simulink model "CPWalker_NAO_simulation"  (R2021b)
settings: Solver=FixedStepDiscrete  StartTime=0.0  StopTime=inf  FixedStep=0.01  RelTol=1e-3
libraries: slrealtimeutilitieslib x1, slrealtimeiplib x1, dspnetwork x1
settings Model: Creator=Julio Lora  LastModifiedBy=mtmau
settings SolverCC: AlgebraicLoopSolver=TrustRegion
settings DataIOCC: ReturnWorkspaceOutputs=off
settings DebuggingCC: SFMachineParentedDataDiag=warning  ArithmeticOperatorsInVariantConditions=warning
settings SFSimCC: SimUseLocalCustomCode=off  CustomCodeUndefinedFunction=UseInterfaceOnly
settings RTWCC: RTWUseLocalCustomCode=off

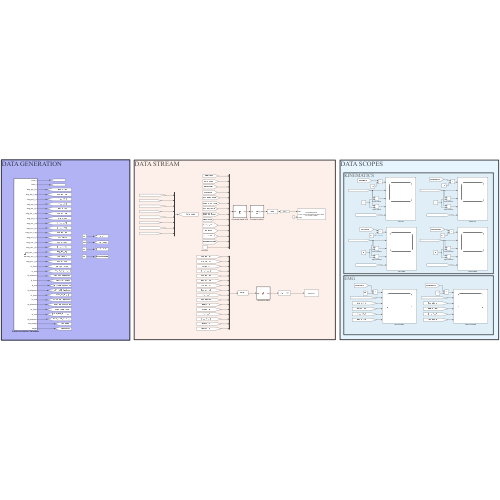
[thumbnail: Simulink's stored preview of the top-level diagram]
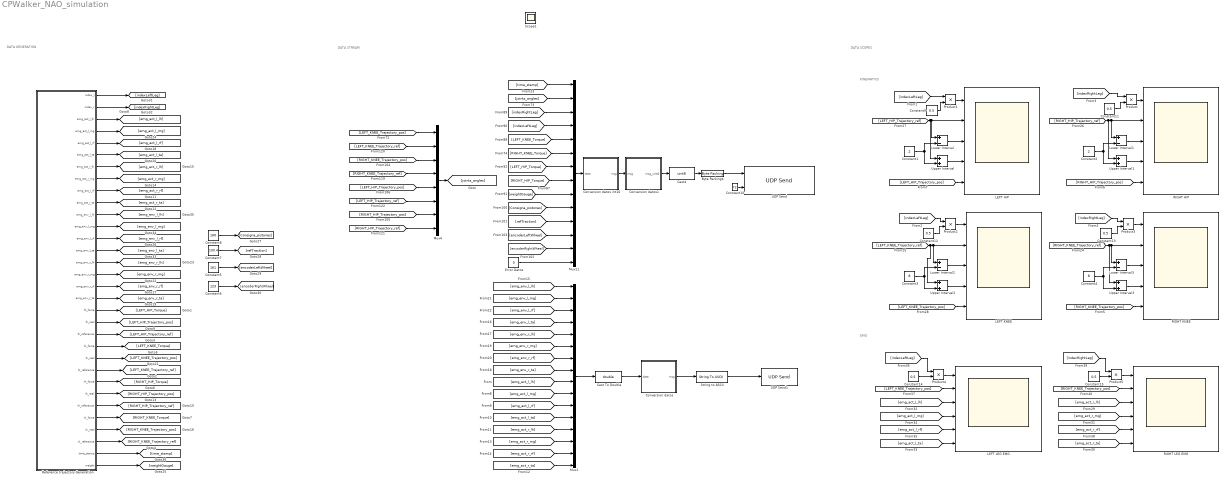
== system CPWalker_NAO_simulation ==
  note: DATA SCOPES
  note: DATA STREAM
  note: DATA GENERATION
  note: KINEMATICS
  note: EMG
  Byte Packing4 : slrealtimeutilitieslib/Byte Packing  MaskPackedDataType=uint8  MaskUnpackedDataTypes={'uint8'}  MaskAlignment=1
  Cast To Double : DataTypeConversion  OutDataTypeStr=double
  Cast4 : DataTypeConversion  OutDataTypeStr=uint8
  Constant1 : Constant  Value=2
  Constant10 : Constant  Value=72
  Constant{9,11..15} (6 alike) : Constant  Value=0.5
  Constant2 : Constant  Value=2
  Constant3 : Constant  Value=8
  Constant4 : Constant  Value=8
  Constant5 : Constant  Value=161
  Constant6 : Constant  Value=123
  Constant7 : Constant  Value=100.4
  Constant8 : Constant  Value=100
  Conversion datos : MATLAB Function  TreatAsAtomicUnit=on
  Conversion datos int16 : MATLAB Function  TreatAsAtomicUnit=on
  Conversion datos1 : MATLAB Function  TreatAsAtomicUnit=on
  Error Datos : Constant  Value=0
  LEFT HIP : Scope  NumInputPorts=5
  LEFT KNEE : Scope  NumInputPorts=5
  LEFT LEG EMG : Scope  NumInputPorts=6
  Lower Interval{,1..3} (4 alike) : Sum  Inputs=+-
  Mux1 : Mux  Inputs=16
  Mux11 : Mux  Inputs=14
  Mux4 : Mux  Inputs=8
  Product{,1..5} (6 alike) : Product
  RIGHT HIP : Scope  NumInputPorts=5
  RIGHT KNEE : Scope  NumInputPorts=5
  RIGHT LEG EMG : Scope  NumInputPorts=6
  Reference trajectory Generation : MATLAB Function  TreatAsAtomicUnit=on
  String to ASCII : StringToASCII  OutputVectorSize=300
  UDP Send : slrealtimeiplib/UDP Send  useHostTargetConn=on  toAddress=127.0.0.1  toPort=10000  sampleTime=-1  ipAddress='127.0.0.1'  localPort=4010
      settings: SourceProductBaseCode=XP
  UDP Send1 : dspnetwork/UDP Send  remoteURL='127.0.0.1'  remotePort=20000  localURL='0.0.0.0'  localPortSource=Automatically determine  localPort=-1  sendBufferSize=200000  sampletime=-1  blockPlatform=[]  separateLengthPort=0
  Upper Interval{,1..3} (4 alike) : Sum
  Scope1 : Scope
  wires:
  Reference trajectory Generation/29(rk_real) -> [RIGHT_KNEE_Trajectory_pos]
  Reference trajectory Generation/26(rh_real) -> [RIGHT_HIP_Trajectory_pos]
  Reference trajectory Generation/20(lh_real) -> [LEFT_HIP_Trajectory_pos]
  Reference trajectory Generation/2(index_r) -> [indexRightLeg]
  Reference trajectory Generation/1(index_l) -> [indexLeftLeg]
  Reference trajectory Generation/23(lk_real) -> [LEFT_KNEE_Trajectory_pos]
  Reference trajectory Generation/24(lk_reference) -> [LEFT_KNEE_Trajectory_ref]
  [LEFT_KNEE_Trajectory_pos] -> Mux4/1
  [LEFT_HIP_Trajectory_pos] -> Mux4/5
  [RIGHT_HIP_Trajectory_ref] -> Mux4/8
  [RIGHT_HIP_Trajectory_pos] -> Mux4/7
  [LEFT_HIP_Trajectory_ref] -> Mux4/6
  [RIGHT_KNEE_Trajectory_ref] -> Mux4/4
  [RIGHT_KNEE_Trajectory_pos] -> Mux4/3
  Constant5/1 -> [encoderLeftWheel]
  Constant6/1 -> [encoderRightWheel]
  Constant7/1 -> [refTraction]
  [LEFT_KNEE_Trajectory_ref] -> Mux4/2
  Constant8/1 -> [Consigna_pistones]
  Reference trajectory Generation/27(rh_reference) -> [RIGHT_HIP_Trajectory_ref]
  Mux4/1 -> [joints_angles]
  Reference trajectory Generation/32(weight) -> [weightGauge]
  Reference trajectory Generation/30(rk_reference) -> [RIGHT_KNEE_Trajectory_ref]
  Reference trajectory Generation/21(lh_reference) -> [LEFT_HIP_Trajectory_ref]
  Reference trajectory Generation/19(lh_force) -> [LEFT_HIP_Torque]
  Reference trajectory Generation/22(lk_force) -> [LEFT_KNEE_Torque]
  Reference trajectory Generation/25(rh_force) -> [RIGHT_HIP_Torque]
  Reference trajectory Generation/28(rk_force) -> [RIGHT_KNEE_Torque]
  [time_stamp] -> Mux11/1
  [LEFT_KNEE_Torque] -> Mux11/5
  Conversion datos int16/1(msg) -> Conversion datos1/1(msg)
  [RIGHT_KNEE_Torque] -> Mux11/6
  [weightGauge] -> Mux11/9
  [RIGHT_HIP_Torque] -> Mux11/8
  Error Datos/1 -> Mux11/14
  Cast4/1 -> Byte Packing4/1
  [LEFT_HIP_Torque] -> Mux11/7
  [encoderLeftWheel] -> Mux11/12
  [refTraction] -> Mux11/11
  [joints_angles] -> Mux11/2
  Conversion datos1/1(msg_uint8) -> Cast4/1
  [encoderRightWheel] -> Mux11/13
  Constant10/1 -> UDP Send/2
  Byte Packing4/1 -> UDP Send/1
  Mux11/1 -> Conversion datos int16/1(data)
  [Consigna_pistones] -> Mux11/10
  Reference trajectory Generation/3(emg_act_l_lh) -> [emg_act_l_lh]
  Reference trajectory Generation/4(emg_act_l_mg) -> [emg_act_l_mg]
  Reference trajectory Generation/5(emg_act_l_rf) -> [emg_act_l_rf]
  Reference trajectory Generation/6(emg_act_l_ta) -> [emg_act_l_ta]
  Reference trajectory Generation/7(emg_act_r_lh) -> [emg_act_r_lh]
  Reference trajectory Generation/8(emg_act_r_mg) -> [emg_act_r_mg]
  Reference trajectory Generation/9(emg_act_r_rf) -> [emg_act_r_rf]
  Reference trajectory Generation/10(emg_act_r_ta) -> [emg_act_r_ta]
  Reference trajectory Generation/11(emg_env_l_lh) -> [emg_env_l_lh]
  Reference trajectory Generation/12(emg_env_l_mg) -> [emg_env_l_mg]
  Reference trajectory Generation/13(emg_env_l_rf) -> [emg_env_l_rf]
  Reference trajectory Generation/14(emg_env_l_ta) -> [emg_env_l_ta]
  Reference trajectory Generation/15(emg_env_r_lh) -> [emg_env_r_lh]
  Reference trajectory Generation/16(emg_env_r_mg) -> [emg_env_r_mg]
  Reference trajectory Generation/17(emg_env_r_rf) -> [emg_env_r_rf]
  Reference trajectory Generation/18(emg_env_r_ta) -> [emg_env_r_ta]
  Mux1/1 -> Cast To Double/1
  [emg_env_l_lh] -> Mux1/1
  [emg_env_l_mg] -> Mux1/2
  [emg_env_l_rf] -> Mux1/3
  [emg_env_l_ta] -> Mux1/4
  [emg_env_r_lh] -> Mux1/5
  [emg_env_r_mg] -> Mux1/6
  [emg_env_r_rf] -> Mux1/7
  [emg_env_r_ta] -> Mux1/8
  [emg_act_l_lh] -> Mux1/9
  [emg_act_l_mg] -> Mux1/10
  [emg_act_l_rf] -> Mux1/11
  [emg_act_l_ta] -> Mux1/12
  [emg_act_r_lh] -> Mux1/13
  [emg_act_r_mg] -> Mux1/14
  [emg_act_r_rf] -> Mux1/15
  [emg_act_r_ta] -> Mux1/16
  Cast To Double/1 -> Conversion datos/1(data)
  String to ASCII/1 -> UDP Send1/1
  Conversion datos/1(msg) -> String to ASCII/1
  Reference trajectory Generation/31(time_stamp) -> [time_stamp]
  [emg_act_l_rf] -> LEFT LEG EMG/5
  [emg_act_l_ta] -> LEFT LEG EMG/6
  [emg_act_l_lh] -> LEFT LEG EMG/3
  [emg_act_l_mg] -> LEFT LEG EMG/4
  [LEFT_KNEE_Trajectory_pos] -> LEFT LEG EMG/2
  [indexLeftLeg] -> Mux11/4
  [indexRightLeg] -> Mux11/3
  Constant1/1 -> Lower Interval/2, Upper Interval/2
  Lower Interval/1 -> LEFT HIP/3
  Upper Interval/1 -> LEFT HIP/4
  Upper Interval1/1 -> RIGHT HIP/4
  Lower Interval1/1 -> RIGHT HIP/3
  Constant2/1 -> Lower Interval1/2, Upper Interval1/2
  Upper Interval2/1 -> LEFT KNEE/4
  Lower Interval2/1 -> LEFT KNEE/3
  Constant3/1 -> Lower Interval2/2, Upper Interval2/2
  Upper Interval3/1 -> RIGHT KNEE/4
  Lower Interval3/1 -> RIGHT KNEE/3
  Constant4/1 -> Lower Interval3/2, Upper Interval3/2
  [LEFT_KNEE_Trajectory_pos] -> LEFT KNEE/5
  [LEFT_KNEE_Trajectory_ref] -> Upper Interval2/1, LEFT KNEE/2, Lower Interval2/1
  [RIGHT_KNEE_Trajectory_pos] -> RIGHT KNEE/5
  [RIGHT_KNEE_Trajectory_ref] -> Upper Interval3/1, RIGHT KNEE/2, Lower Interval3/1
  [LEFT_HIP_Trajectory_pos] -> LEFT HIP/5
  [LEFT_HIP_Trajectory_ref] -> Upper Interval/1, LEFT HIP/2, Lower Interval/1
  [RIGHT_HIP_Trajectory_pos] -> RIGHT HIP/5
  [RIGHT_HIP_Trajectory_ref] -> Upper Interval1/1, Lower Interval1/1, RIGHT HIP/2
  [emg_act_r_ta] -> RIGHT LEG EMG/6
  [emg_act_r_lh] -> RIGHT LEG EMG/3
  [emg_act_r_mg] -> RIGHT LEG EMG/4
  [RIGHT_KNEE_Trajectory_pos] -> RIGHT LEG EMG/2
  [emg_act_r_rf] -> RIGHT LEG EMG/5
  Constant11/1 -> Product/2
  Product/1 -> RIGHT HIP/1
  [indexRightLeg] -> Product/1
  Constant9/1 -> Product1/2
  Product1/1 -> LEFT HIP/1
  [indexLeftLeg] -> Product1/1
  Constant12/1 -> Product2/2
  Product2/1 -> LEFT KNEE/1
  [indexLeftLeg] -> Product2/1
  Constant13/1 -> Product3/2
  Product3/1 -> RIGHT KNEE/1
  [indexRightLeg] -> Product3/1
  Constant14/1 -> Product4/2
  Product4/1 -> LEFT LEG EMG/1
  [indexLeftLeg] -> Product4/1
  Constant15/1 -> Product5/2
  Product5/1 -> RIGHT LEG EMG/1
  [indexRightLeg] -> Product5/1

== matlab function CPWalker_NAO_simulation/Conversion datos1 ==
  data: msg input; msg_uint8 output
function msg_uint8 = fcn(msg)

msg_uint8 = zeros(1,72);
index = 1;

% Time data
msg_converted = typecast(int32(msg(1)),'uint8').';
msg_uint8(index) = msg_converted(4);
index = index + 1;
msg_uint8(index) = msg_converted(3);
index = index + 1;
msg_uint8(index) = msg_converted(2);
index = index + 1;
msg_uint8(index) = msg_converted(1);
index = index + 1;

% Joints data
for i=2:17
    msg_converted = typecast(int16(msg(i)),'uint8').';
    msg_uint8(index) = msg_converted(1);
    index = index + 1;
    msg_uint8(index) = msg_converted(2);
    index = index + 1;
end 

% Leg index
msg_converted = typecast(uint8(msg(18)),'uint8').';
msg_uint8(index) = msg_converted(1);
index = index + 1;
msg_converted = typecast(uint8(msg(19)),'uint8').';
msg_uint8(index) = msg_converted(1);
index = index + 1;

% Joint torques and weight
for i=20:30
    msg_converted = typecast(int16(msg(i)),'uint8').';
    msg_uint8(index) = msg_converted(1);
    index = index + 1;
    msg_uint8(index) = msg_converted(2);
    index = index + 1;
end 

% Pistons ref
msg_converted = typecast(int16(msg(31)),'uint8').';
msg_uint8(index) = msg_converted(1);
index = index + 1;

% Traction
for i=32:36
    msg_converted = typecast(int16(msg(i)),'uint8').';
    msg_uint8(index) = msg_converted(1);
    index = index + 1;
    msg_uint8(index) = msg_converted(2);
    index = index + 1;
end

% Data error
msg_converted = typecast(int16(msg(37)),'uint8').';
msg_uint8(index) = msg_converted(1);


end

== matlab function CPWalker_NAO_simulation/Conversion datos int16 ==
  data: data input; msg output
function msg = fcn(data)
%% Test
% Esta función reordena los datos registrados y generados por la
% plataforma. Los datos enviados son :
% - Posiciones reales de las 4 articulaciones (medidas por los
%   potenciómetros).
% - Posiciones de referencia (generadas por el generador de trayectorias).
msg = zeros(1,37);

% for i = 1:length(data)
%     data(i) = -0.1;
% end

% Angles Reference and potentiometer
% Time
msg(1) = uint32(data(1) * 1000);
% Left knee pot:
[msg(2), msg(3)] = divideNumber(data(2));
% Left knee ref:
[msg(4), msg(5)] = divideNumber(data(3));
% Right knee pot:
[msg(6), msg(7)] = divideNumber(data(4));
% Right knee ref:
[msg(8), msg(9)] = divideNumber(data(5));
% Left hip pot:
[msg(10), msg(11)] = divideNumber(data(6));
% Left hip ref:
[msg(12), msg(13)] = divideNumber(data(7));
% Right hip pot:
[msg(14), msg(15)] = divideNumber(data(8));
% Right hip ref:
[msg(16), msg(17)] = divideNumber(data(9));
% Leg Gait Index
msg(18) = uint8(fix(data(10)));
msg(19) = uint8(fix(data(11)));
% Leg Torques
[msg(20), msg(21)] = divideNumber(data(12));
[msg(22), msg(23)] = divideNumber(data(13));
[msg(24), msg(25)] = divideNumber(data(14));
[msg(26), msg(27)] = divideNumber(data(15));
% Weigth Gauge
[msg(28), msg(29)] = divideNumber(data(16));
% Pistons control
msg(30)= int8(data(17));
% Traction reference
[msg(31), msg(32)] = divideNumber(data(18));
% Encoders velocity
[msg(33), msg(34)] = divideNumber(data(19));
[msg(35), msg(36)] = divideNumber(data(20));
% Error
msg(37) = int8(int8(fix(data(21))));
    


end
    
% Dividir numero en su valor entero y decimal
function [interger, decimal] = divideNumber(number)
    interger = int16(fix(number));
     if (number > -1 && number < 0)
         interger = int16(32767);
         decimal = int16((abs(number))*1000);
     else
         decimal = int16((abs(number) - double(abs(interger)))*1000);
     end

end

== matlab function CPWalker_NAO_simulation/Conversion datos ==
  data: data input; msg output
function msg = fcn(data)
%% Test
% Esta función reordena los datos registrados y generados por la
% plataforma. Los datos enviados son :
% - Posiciones reales de las 4 articulaciones (medidas por los
%   potenciómetros).
% - Posiciones de referencia (generadas por el generador de trayectorias).


emg_env= [data(1), data(2), data(3), data(4), data(5), data(6), data(7), data(8)];
emg_act = [data(9), data(10), data(11), data(12), data(13), data(14), data(15), data(16)];

msg = convertCharsToStrings(['{' '"emg": [' sprintf(' %.11f', data(1)) ' ,' sprintf(' %.11f', data(2)) ' ,' sprintf(' %.11f', data(3)) ' ,' sprintf(' %.11f', data(4)) ' ,' sprintf(' %.11f', data(5)) ' ,' sprintf(' %.11f', data(6)) ' ,' sprintf(' %.11f', data(7)) ' ,' sprintf(' %.11f', data(8)) '], "binary_activation_values": [' sprintf('%.0f', data(9)) ' ,' sprintf('%.0f', data(10)) ' ,' sprintf('%.0f', data(11)) ' ,' sprintf('%.0f', data(12)) ' ,' sprintf('%.0f', data(13)) ' ,' sprintf('%.0f', data(14)) ' ,' sprintf('%.0f', data(15)) ' ,' sprintf('%.0f', data(16)) '], "threshold_errors": [4, 4, 4, 4, 4, 4, 4, 4], "threshold_values": [0,0,0,0,0,0,0,0]}']);
% msg = convertCharsToStrings('{"emg": [1,2,3,4,5,6,7,8], "binary_activation_values":[1,1,1,1,1,1,1,1],"threshold_errors": [4, 4, 4, 4, 4, 4, 4, 4], "threshold_values": [0,0,0,0,0,0,0,0]}');
end

== matlab function CPWalker_NAO_simulation/Reference trajectory Generation ==
  settings: updateMethod=DISCRETE
  data: index_l output; index_r output; emg_act_l_lh output; emg_act_l_mg output; emg_act_l_rf output; emg_act_l_ta output; emg_act_r_lh output; emg_act_r_mg output; emg_act_r_rf output; emg_act_r_ta output; emg_env_l_lh output; emg_env_l_mg output; emg_env_l_rf output; emg_env_l_ta output; emg_env_r_lh output; emg_env_r_mg output; emg_env_r_rf output; emg_env_r_ta output; lh_force output; lh_real output; lh_reference output; lk_force output; lk_real output; lk_reference output; rh_force output; rh_real output; rh_reference output; rk_force output; rk_real output; rk_reference output; time_stamp output; weight output
function [index_l, index_r,emg_act_l_lh, emg_act_l_mg, emg_act_l_rf, emg_act_l_ta, emg_act_r_lh, emg_act_r_mg, emg_act_r_rf, emg_act_r_ta, emg_env_l_lh, emg_env_l_mg, emg_env_l_rf, emg_env_l_ta, emg_env_r_lh, emg_env_r_mg, emg_env_r_rf, emg_env_r_ta, lh_force, lh_real, lh_reference, lk_force, lk_real, lk_reference, rh_force, rh_real, rh_reference, rk_force, rk_real, rk_reference, time_stamp, weight]= fcn()
persistent initialize   % Initilize variables
persistent index_l_session index_r_session emg_act_l_lh_session emg_act_l_mg_session emg_act_l_rf_session emg_act_l_ta_session emg_act_r_lh_session emg_act_r_mg_session emg_act_r_rf_session emg_act_r_ta_session emg_env_l_lh_session emg_env_l_mg_session emg_env_l_rf_session emg_env_l_ta_session emg_env_r_lh_session emg_env_r_mg_session emg_env_r_rf_session emg_env_r_ta_session lh_force_session lh_real_session lh_reference_session lk_force_session lk_real_session lk_reference_session rh_force_session rh_real_session rh_reference_session rk_force_session rk_real_session rk_reference_session time_stamp_session weight_session;
persistent count        % Variable used to loop through the data
persistent start_gait   % True when exoskeleton start to move 
persistent last_time    % Last moment when the control setpoints where updated 

%% Import session data
if isempty(initialize)
    %% Select file
    file_name = "Session_16.mat";
    initialize = 1;
    count = 0;
    %% Load data   
    % Get EMG data
    emg_act_l_lh_session = load(file_name,'emg_act_l_lh'); 
    emg_act_l_mg_session = load(file_name,'emg_act_l_mg');
    emg_act_l_rf_session = load(file_name,'emg_act_l_rf');
    emg_act_l_ta_session = load(file_name,'emg_act_l_ta');
    emg_act_r_lh_session = load(file_name,'emg_act_r_lh');
    emg_act_r_mg_session = load(file_name,'emg_act_r_mg');
    emg_act_r_rf_session = load(file_name,'emg_act_r_rf');
    emg_act_r_ta_session = load(file_name,'emg_act_r_ta');
    emg_env_l_lh_session = load(file_name,'emg_env_l_lh');
    emg_env_l_mg_session = load(file_name,'emg_env_l_mg');
    emg_env_l_rf_session = load(file_name,'emg_env_l_rf');
    emg_env_l_ta_session = load(file_name,'emg_env_l_ta');
    emg_env_r_lh_session = load(file_name,'emg_env_r_lh');
    emg_env_r_mg_session = load(file_name,'emg_env_r_mg');
    emg_env_r_rf_session = load(file_name,'emg_env_r_rf');
    emg_env_r_ta_session = load(file_name,'emg_env_r_ta');
    
    % Smooth EGM data
    emg_env_l_lh_session.emg_env_l_lh = smoothdata(emg_env_l_lh_session.emg_env_l_lh,'gaussian',20);
    emg_env_l_mg_session.emg_env_l_mg = smoothdata(emg_env_l_mg_session.emg_env_l_mg,'gaussian',20);
    emg_env_l_rf_session.emg_env_l_rf = smoothdata(emg_env_l_rf_session.emg_env_l_rf,'gaussian',20);
    emg_env_l_ta_session.emg_env_l_ta = smoothdata(emg_env_l_ta_session.emg_env_l_ta,'gaussian',20);
    emg_env_r_lh_session.emg_env_r_lh = smoothdata(emg_env_r_lh_session.emg_env_r_lh,'gaussian',20);
    emg_env_r_mg_session.emg_env_r_mg = smoothdata(emg_env_r_mg_session.emg_env_r_mg,'gaussian',20);
    emg_env_r_rf_session.emg_env_r_rf = smoothdata(emg_env_r_rf_session.emg_env_r_rf,'gaussian',20);
    emg_env_r_ta_session.emg_env_r_ta = smoothdata(emg_env_r_ta_session.emg_env_r_ta,'gaussian',20);
    
    % Get kinematics and kinetic data
    lh_force_session = load(file_name,'lh_force');
    lh_real_session = load(file_name,'lh_real');
    lh_reference_session = load(file_name,'lh_reference');
    lk_force_session = load(file_name,'lk_force');
    lk_real_session = load(file_name,'lk_real');
    lk_reference_session = load(file_name,'lk_reference');
    rh_force_session = load(file_name,'rh_force');
    rh_real_session = load(file_name,'rh_real');
    rh_reference_session = load(file_name,'rh_reference');
    rk_force_session = load(file_name,'rk_force');
    rk_real_session = load(file_name,'rk_real');
    rk_reference_session = load(file_name,'rk_reference');
    time_stamp_session = load(file_name,'time_stamp');
    weight_session = load(file_name,'weight');
end

%% Generate gait index.
if isempty(index_r_session) 
    index_r_session = 71;
end
if isempty(index_l_session)
    index_l_session = 0;
end
if isempty(start_gait)
    start_gait = 0;
end
if isempty(last_time)
    last_time=0;
end

% Number of samples in session
n = length(time_stamp_session.time_stamp(:));

% Calculate delta time increment according to session data:
% (Constants obtained from CPWaker Sessions Database)
delta_angle = 0.42426;
ROM = 100/100;
leg_length = 0.8;
wheel_r = 17.5 /2;
linear_velocity = 0.954585;
delta_time = round((delta_angle * ROM) * leg_length / (linear_velocity * wheel_r)*100)/100;

% Update index
i = mod(count,n);
if i == 0
    i = 1;
end
if (start_gait == 0 && i > 1 && rh_reference_session.rh_reference(i-1) ~= rh_reference_session.rh_reference(i))
   index_r_session = 72;
   index_l_session = 171;
   start_gait = 1;
else
    if (start_gait == 0)
        % Initial values
        index_r_session = 72;
        index_l_session = 171;
        last_time = time_stamp_session.time_stamp(i);
    elseif (rh_reference_session.rh_reference(i-1) ~= rh_reference_session.rh_reference(i) && (time_stamp_session.time_stamp(i) - last_time >= 1000 * delta_time)) 
        % Increase index
        index_r_session = mod(index_r_session + round(time_stamp_session.time_stamp(i) - last_time)/(1000 * delta_time), 201);
        index_l_session = mod(index_l_session + round(time_stamp_session.time_stamp(i) - last_time)/(1000 * delta_time), 201);
        % Never index = 0
        if (index_r_session == 0) 
            index_r_session = 1;
        end
        if (index_l_session == 0) 
            index_l_session = 1;
        end
        % Update last time stamp
        last_time = time_stamp_session.time_stamp(i);
    end
end


%% Update data
emg_act_l_lh = emg_act_l_lh_session.emg_act_l_lh(i); 
emg_act_l_mg = emg_act_l_mg_session.emg_act_l_mg(i);
emg_act_l_rf = emg_act_l_rf_session.emg_act_l_rf(i);
emg_act_l_ta = emg_act_l_ta_session.emg_act_l_ta(i);
emg_act_r_lh = emg_act_r_lh_session.emg_act_r_lh(i);
emg_act_r_mg = emg_act_r_mg_session.emg_act_r_mg(i);
emg_act_r_rf = emg_act_r_rf_session.emg_act_r_rf(i);
emg_act_r_ta = emg_act_r_ta_session.emg_act_r_ta(i);
emg_env_l_lh = emg_env_l_lh_session.emg_env_l_lh(i);
emg_env_l_mg = emg_env_l_mg_session.emg_env_l_mg(i);
emg_env_l_rf = emg_env_l_rf_session.emg_env_l_rf(i);
emg_env_l_ta = emg_env_l_ta_session.emg_env_l_ta(i);
emg_env_r_lh = emg_env_r_lh_session.emg_env_r_lh(i);
emg_env_r_mg = emg_env_r_mg_session.emg_env_r_mg(i);
emg_env_r_rf = emg_env_r_rf_session.emg_env_r_rf(i);
emg_env_r_ta = emg_env_r_ta_session.emg_env_r_ta(i);
lh_force = lh_force_session.lh_force(i);
lh_real = lh_real_session.lh_real(i);
lh_reference = lh_reference_session.lh_reference(i);
lk_force = lk_force_session.lk_force(i);
lk_real = lk_real_session.lk_real(i);
lk_reference = lk_reference_session.lk_reference(i);
rh_force = rh_force_session.rh_force(i);
rh_real = rh_real_session.rh_real(i);
rh_reference = rh_reference_session.rh_reference(i);
rk_force = rk_force_session.rk_force(i);
rk_real = rk_real_session.rk_real(i);
rk_reference = rk_reference_session.rk_reference(i);
time_stamp = time_stamp_session.time_stamp(i);
weight = weight_session.weight(i);
index_l = index_l_session;
index_r = index_r_session;

count = count + 1;

end
